simulink model "bench_thermal_plant"  (R2024b)
settings: Solver=daessc  StartTime=0.0  StopTime=3600  MaxStep=5  RelTol=1e-3
libraries: loco_native_lib x1
settings Model: Creator=BillBeverley  LastModifiedBy=BillBeverley

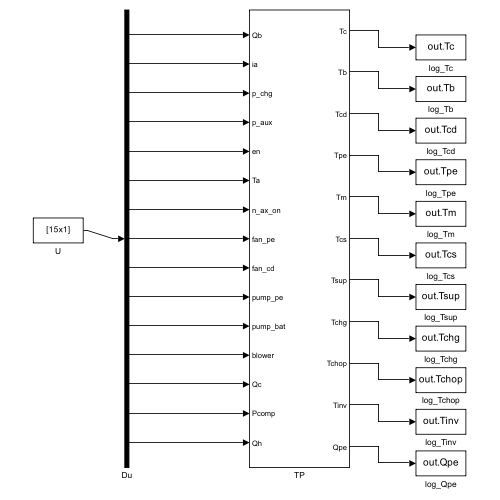
[thumbnail: Simulink's stored preview of the top-level diagram]
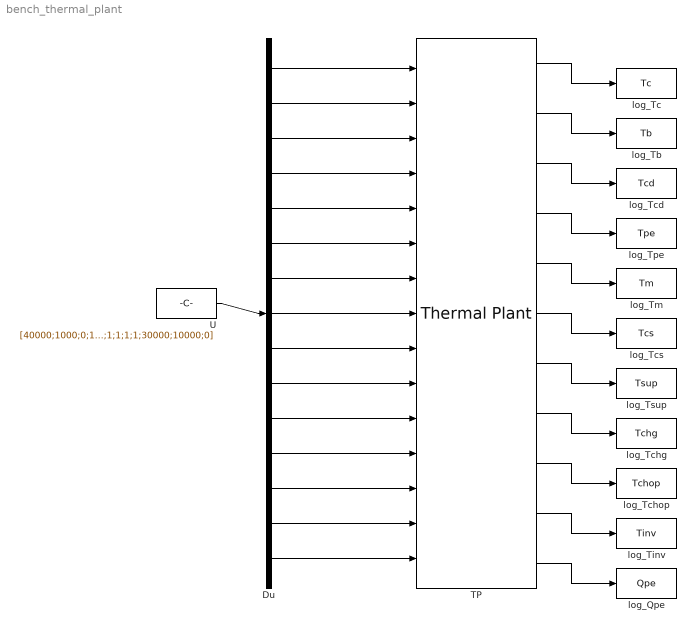
== system bench_thermal_plant ==
  Du : Demux  Outputs=15
  TP : loco_native_lib/Thermal Plant  TH=P.th  f_ram=0.2
  U : Constant  Value=[40000;1000;0;100000;1;313.15;4;1;1;1;1;1;30000;10000;0]
  log_Qpe : ToWorkspace  VariableName=Qpe  SaveFormat=Timeseries  SampleTime=-1
  log_Tb : ToWorkspace  VariableName=Tb  SaveFormat=Timeseries  SampleTime=-1
  log_Tc : ToWorkspace  VariableName=Tc  SaveFormat=Timeseries  SampleTime=-1
  log_Tcd : ToWorkspace  VariableName=Tcd  SaveFormat=Timeseries  SampleTime=-1
  log_Tchg : ToWorkspace  VariableName=Tchg  SaveFormat=Timeseries  SampleTime=-1
  log_Tchop : ToWorkspace  VariableName=Tchop  SaveFormat=Timeseries  SampleTime=-1
  log_Tcs : ToWorkspace  VariableName=Tcs  SaveFormat=Timeseries  SampleTime=-1
  log_Tinv : ToWorkspace  VariableName=Tinv  SaveFormat=Timeseries  SampleTime=-1
  log_Tm : ToWorkspace  VariableName=Tm  SaveFormat=Timeseries  SampleTime=-1
  log_Tpe : ToWorkspace  VariableName=Tpe  SaveFormat=Timeseries  SampleTime=-1
  log_Tsup : ToWorkspace  VariableName=Tsup  SaveFormat=Timeseries  SampleTime=-1
  wires:
  U/1 -> Du/1
  Du/1 -> TP/1
  Du/2 -> TP/2
  Du/3 -> TP/3
  Du/4 -> TP/4
  Du/5 -> TP/5
  Du/6 -> TP/6
  Du/7 -> TP/7
  Du/8 -> TP/8
  Du/9 -> TP/9
  Du/10 -> TP/10
  Du/11 -> TP/11
  Du/12 -> TP/12
  Du/13 -> TP/13
  Du/14 -> TP/14
  Du/15 -> TP/15
  TP/1 -> log_Tc/1
  TP/2 -> log_Tb/1
  TP/3 -> log_Tcd/1
  TP/4 -> log_Tpe/1
  TP/5 -> log_Tm/1
  TP/6 -> log_Tcs/1
  TP/7 -> log_Tsup/1
  TP/8 -> log_Tchg/1
  TP/9 -> log_Tchop/1
  TP/10 -> log_Tinv/1
  TP/11 -> log_Qpe/1
